simulink model "6DOF_model_2"  (R2019b)
settings: Solver=VariableStepAuto  StartTime=0.0  StopTime=10.0  RelTol=1e-3
values from neighbouring files (symbols this model uses):
  altitude = 0    [runFrist.m]
  AR = b^2/S    (= 7.81468427964)    [runFrist.m]
  b = 1.4224    [runFrist.m]
  c_bar = 0.3302    [runFrist.m]
  CDdelta_e = 0    [runFrist.m]
  Cdo = 0.03    [runFrist.m]
  CDq = 0    [runFrist.m]
  Clbeta = -0.12    [runFrist.m]
  Cldelta_a = 0.08    [runFrist.m]
  CLdelta_e = -0.36    [runFrist.m]
  Cldelta_r = 0.105    [runFrist.m]
  Clo = 0    [runFrist.m]
  Clp = -0.26    [runFrist.m]
  CLq = 0    [runFrist.m]
  Clr = 0.14    [runFrist.m]
  Cmalpha = -0.38    [runFrist.m]
  Cmdelta_e = -0.5    [runFrist.m]
  Cmo = 0    [runFrist.m]
  Cmq = -3.6    [runFrist.m]
  Cnbeta = 0.25    [runFrist.m]
  Cndelta_a = 0.06    [runFrist.m]
  Cndelta_r = -0.032    [runFrist.m]
  Cno = 0    [runFrist.m]
  Cnp = 0.022    [runFrist.m]
  Cnr = -0.35    [runFrist.m]
  Cybeta = -0.98    [runFrist.m]
  Cydelta_a = 0    [runFrist.m]
  Cydelta_r = -0.17    [runFrist.m]
  Cyo = 0    [runFrist.m]
  Cyp = 0    [runFrist.m]
  Cyr = 0    [runFrist.m]
  delta = Iz*Ix-Ixz^2    (= 196.36639775)    [runFrist.m]
  g = 9.81    [runFrist.m]
  I1 = Ixz*(Ix-Iy+Iz)    (= 2.56808565)    [runFrist.m]
  I2 = Iy*Iz-Iz^2-Ixz^2    (= -2930845.3888)    [runFrist.m]
  I3 = Ixz^2-Iy*Ix+Ix^2    (= 0.00655162)    [runFrist.m]
  Ix = 0.1147    [runFrist.m]
  Ixz = 0.0015    [runFrist.m]
  Iy = 0.0576    [runFrist.m]
  Iz = 01712    (= 1712)    [runFrist.m]
  m = 1.56    [runFrist.m]
  S = 0.2589    [runFrist.m]
  Thrust = 10    [runFrist.m]
  Uo = 0.01    [runFrist.m]
settings Model: Creator=Tinash  LastModifiedBy=Tinash

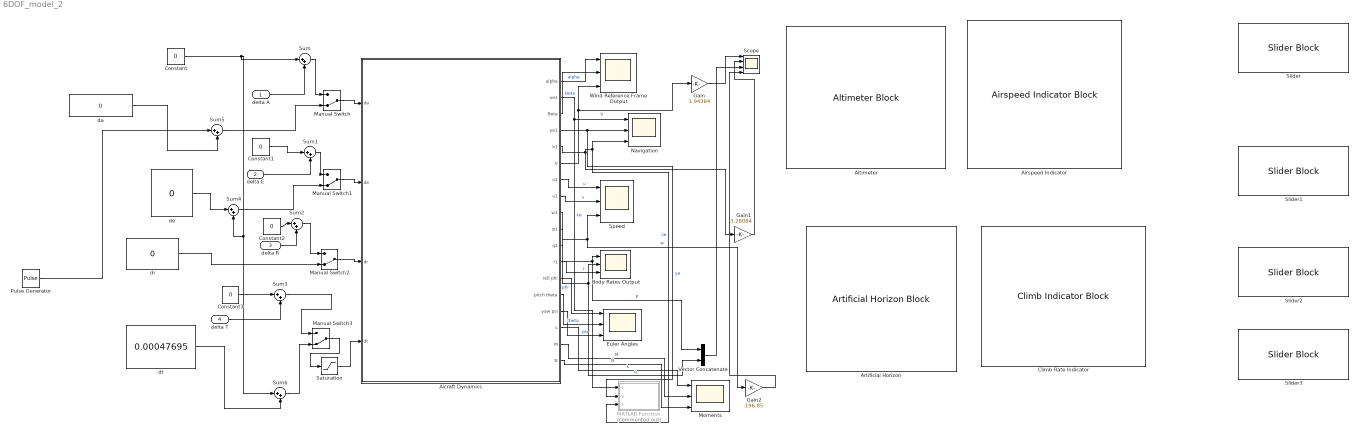
== system 6DOF_model_2 ==
  delta A : Inport
  delta E : Inport  Port=2
  delta R : Inport  Port=3
  delta T : Inport  Port=4
  Aicraft Dynamics : Subsystem
  Airspeed Indicator : AirspeedIndicatorBlock  BlockKeywords=__PRM__SERIALIZED__DATA__:flight instrument,gauge,cockpit,measurement,display,graphics,visualization,dashboard,aircraft,needle,instrumentation,speed,stall speed,maximum speed,max speed,ASI  ScaleMin=0  ScaleMax=100
  Altimeter : AltimeterBlock  BlockKeywords=__PRM__SERIALIZED__DATA__:flight instrument,gauge,cockpit,measurement,indicator,display,graphics,visualization,dashboard,aircraft,needle,instrumentation,altitude,height,height above sea level,altimetry,pressure altitude,atmospheric pressure
  Artificial Horizon : ArtificialHorizonBlock  BlockKeywords=__PRM__SERIALIZED__DATA__:flight instrument,gauge,cockpit,measurement,indicator,display,graphics,visualization,dashboard,aircraft,instrumentation,roll,pitch,attitude,angle,gyro horizon,gyroscope
  Body Rates Output : Scope  NumInputPorts=3
  Climb Rate Indicator : ClimbIndicatorBlock  BlockKeywords=__PRM__SERIALIZED__DATA__:flight instrument,gauge,cockpit,measurement,indicator,display,graphics,visualization,dashboard,aircraft,needle,instrumentation,climb indicator,altitude,sink rate,rate of descent,rate of ascent,vertical speed,variometer,vertical speed indicator,VSI,vertical velocity indicator,VVI,RCDI
  Constant{,1..3} (4 alike) : Constant  Value=0
  Euler Angles : Scope  NumInputPorts=3
  Gain : Gain  Gain=1.94384
  Gain1 : Gain  Gain=3.28084
  Gain2 : Gain  Gain=196.85
  MATLAB Function : MATLAB Function  Commented=on  TreatAsAtomicUnit=on
  Manual Switch{,1..3} (4 alike) : ManualSwitch  CurrentSetting=0
  Moments : Scope  NumInputPorts=3
  Navigation : Scope  NumInputPorts=3
  Pulse Generator : DiscretePulseGenerator  PulseType=Time based  Amplitude=0.1
  Saturation : Saturate  UpperLimit=inf  LowerLimit=-inf
  Scope : Scope  NumInputPorts=4
  Slider : SliderBlock  ScaleMin=-10  ScaleMax=10
  Slider1 : SliderBlock  ScaleMin=-10  ScaleMax=10
  Slider2 : SliderBlock  ScaleMin=-10  ScaleMax=10
  Slider3 : SliderBlock
  Speed : Scope  NumInputPorts=3
  Sum{,1..6} (7 alike) : Sum  Inputs=|++
  Vector Concatenate : Concatenate
  "Wind Reference Frame Output " : Scope  NumInputPorts=3
  da : Constant  Value=0
  de : Constant  Value=0
  dr : Constant  Value=0
  dt : Constant  Value=0.00047695  VectorParams1D=off
  wires:
  Saturation/1 -> Aicraft Dynamics/4(dt)
  Pulse Generator/1 -> Sum5/1
  Aicraft Dynamics/8(v1) -> Speed/2  "v"
  da/1 -> Sum5/2
  de/1 -> Sum4/1
  dt/1 -> Sum6/2
  Constant1/1 -> Sum1/1
  Manual Switch/1 -> Aicraft Dynamics/1(da)
  Sum3/1 -> Manual Switch3/1
  Sum4/1 -> Manual Switch1/2
  Aicraft Dynamics/3(Beta) -> "Wind Reference Frame Output "/2  "Beta"
  Aicraft Dynamics/12(r1) -> Body Rates Output/3  "r"
  Sum2/1 -> Manual Switch2/1
  Constant2/1 -> Sum2/1
  delta T/1 -> Sum3/2
  Sum6/1 -> Manual Switch3/2
  Sum/1 -> Manual Switch/1
  Sum5/1 -> Manual Switch/2
  Aicraft Dynamics/4(ye1) -> MATLAB Function/2(y), Navigation/2  "ye"
  Manual Switch3/1 -> Saturation/1
  Aicraft Dynamics/11(q1) -> Body Rates Output/2, Vector Concatenate/2  "q"
  Manual Switch2/1 -> Aicraft Dynamics/3(dr)
  Constant/1 -> Sum4/2, Sum6/1, Sum/1
  Aicraft Dynamics/9(w1) -> Speed/3, Gain2/1  "w"
  Aicraft Dynamics/10(p1) -> Body Rates Output/1, Vector Concatenate/1  "p"
  delta E/1 -> Sum1/2
  Aicraft Dynamics/15(yaw psi) -> Euler Angles/3  "psi"
  Manual Switch1/1 -> Aicraft Dynamics/2(de)
  Constant3/1 -> Sum3/1
  Aicraft Dynamics/7(u1) -> Speed/1  "u"
  Gain2/1 -> Scope/4
  dr/1 -> Manual Switch2/2
  delta R/1 -> Sum2/2
  Aicraft Dynamics/2(xe1) -> MATLAB Function/1(x), Navigation/1  "xe"
  delta A/1 -> Sum/2
  Aicraft Dynamics/6(V) -> Gain/1, "Wind Reference Frame Output "/3  "V"
  Aicraft Dynamics/1(alpha) -> "Wind Reference Frame Output "/1  "alpha"
  Sum1/1 -> Manual Switch1/1
  Aicraft Dynamics/13(roll phi) -> Euler Angles/1  "phi"
  Aicraft Dynamics/5(h1) -> MATLAB Function/3(z), Navigation/3, Gain1/1  "ze"
  Vector Concatenate/1 -> Scope/3
  Gain/1 -> Scope/1
  Gain1/1 -> Scope/2
  Aicraft Dynamics/14(pitch theta) -> Euler Angles/2  "theta"
  Aicraft Dynamics/16(L) -> Moments/1  "L"
  Aicraft Dynamics/17(M) -> Moments/2  "M"
  Aicraft Dynamics/18(N) -> Moments/3  "N"

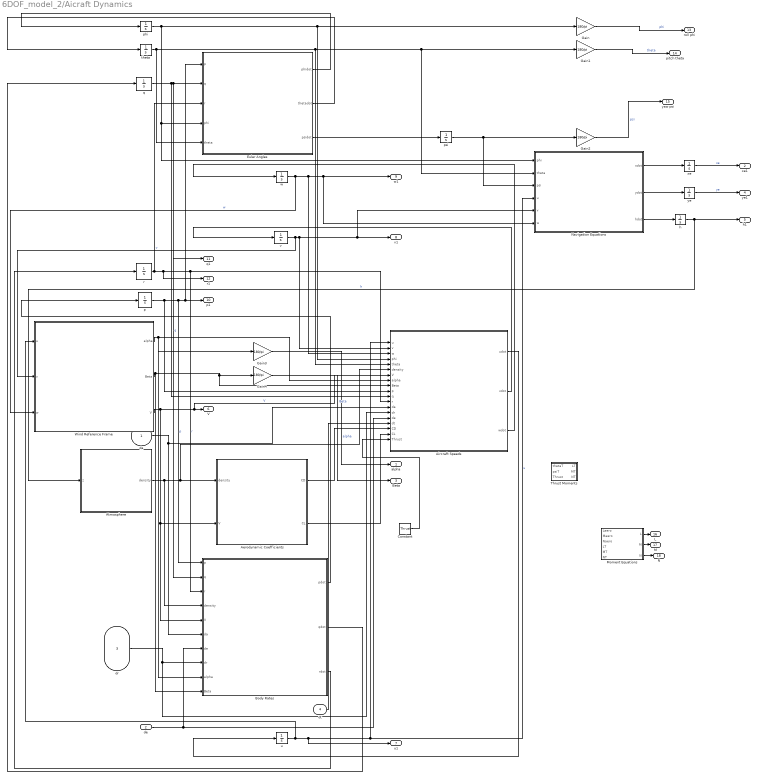
== system 6DOF_model_2/Aicraft Dynamics ==
  da : Inport
  de : Inport  Port=2
  dr : Inport  Port=3
  dt : Inport  Port=4
  Aerodynamic Coefficients : MATLAB Function  TreatAsAtomicUnit=on
  Aircraft Speeds : MATLAB Function  TreatAsAtomicUnit=on
  Atmosphere : MATLAB Function  TreatAsAtomicUnit=on
  Body Rates : MATLAB Function  TreatAsAtomicUnit=on
  Constant : Constant  Value=Thrust
  Euler Angles : MATLAB Function  TreatAsAtomicUnit=on
  Gain{,1..4} (5 alike) : Gain  Gain=180/pi
  Moment Equations : MATLAB Function  TreatAsAtomicUnit=on
  Navigation Equations : MATLAB Function  TreatAsAtomicUnit=on
  Thrust Moments : MATLAB Function  TreatAsAtomicUnit=on
  Wind Reference Frame : MATLAB Function  TreatAsAtomicUnit=on
  h : Integrator  InitialCondition=altitude  LimitOutput=on  LowerSaturationLimit=0
  p : Integrator
  phi : Integrator  LimitOutput=on  UpperSaturationLimit=2*pi  LowerSaturationLimit=0
  psi : Integrator  LimitOutput=on  UpperSaturationLimit=2*pi  LowerSaturationLimit=0
  q : Integrator
  r : Integrator
  theta : Integrator  LimitOutput=on  UpperSaturationLimit=0.9999*(pi/2)  LowerSaturationLimit=-0.99999*(pi/2)
  u : Integrator  InitialCondition=Uo  LimitOutput=on  LowerSaturationLimit=0.000000001
  v : Integrator
  w : Integrator
  xe : Integrator
  ye : Integrator
  alpha : Outport
  xe1 : Outport  Port=2
  Beta : Outport  Port=3
  ye1 : Outport  Port=4
  h1 : Outport  Port=5
  V : Outport  Port=6
  u1 : Outport  Port=7
  v1 : Outport  Port=8
  w1 : Outport  Port=9
  p1 : Outport  Port=10
  q1 : Outport  Port=11
  r1 : Outport  Port=12
  roll phi : Outport  Port=13
  pitch theta : Outport  Port=14
  yaw psi : Outport  Port=15
  L : Outport  Port=16
  M : Outport  Port=17
  N : Outport  Port=18
  wires:
  Gain4/1 -> Beta/1  "Beta"
  q/1 -> Euler Angles/2(q), q1/1, Body Rates/2(q), Aircraft Speeds/11(q)  "q"
  ye/1 -> ye1/1  "ye"
  r/1 -> Body Rates/3(r), Aircraft Speeds/12(r), r1/1, Euler Angles/3(r)  "r"
  Gain3/1 -> alpha/1  "alpha"
  xe/1 -> xe1/1  "xe"
  Body Rates/3(rdot) -> r/1
  Body Rates/2(qdot) -> q/1
  Euler Angles/3(psidot) -> psi/1
  Aircraft Speeds/3(wdot) -> w/1
  Euler Angles/2(thetadot) -> theta/1
  v/1 -> Navigation Equations/5(v), v1/1, Aircraft Speeds/2(v), Wind Reference Frame/2(v)  "v"
  Euler Angles/1(phidot) -> phi/1
  Body Rates/1(pdot) -> p/1
  Wind Reference Frame/1(alpha) -> Gain3/1, Aircraft Speeds/8(alpha), Body Rates/9(alpha)
  Aerodynamic Coefficients/2(CL) -> Aircraft Speeds/18(CL)
  dt/1 -> Aircraft Speeds/16(dt)
  Navigation Equations/2(ydot) -> ye/1
  theta/1 -> Navigation Equations/2(theta), Gain1/1, Aircraft Speeds/5(theta), Euler Angles/5(theta)
  psi/1 -> Gain2/1, Navigation Equations/3(psi)
  phi/1 -> Navigation Equations/1(phi), Euler Angles/4(phi), Aircraft Speeds/4(phi), Gain/1
  Navigation Equations/1(xdot) -> xe/1
  Aircraft Speeds/2(vdot) -> v/1
  Aircraft Speeds/1(udot) -> u/1
  Aerodynamic Coefficients/1(CD) -> Aircraft Speeds/17(CD)
  Navigation Equations/3(hdot) -> h/1
  da/1 -> Body Rates/6(da), Aircraft Speeds/13(da)
  w/1 -> Navigation Equations/6(w), w1/1, Aircraft Speeds/3(w), Wind Reference Frame/3(w)  "w"
  p/1 -> Euler Angles/1(p), p1/1, Body Rates/1(p), Aircraft Speeds/10(p)  "p"
  u/1 -> Aircraft Speeds/1(u), Navigation Equations/4(u), u1/1, Wind Reference Frame/1(u)  "u"
  h/1 -> Atmosphere/1(z), h1/1  "h"
  de/1 -> Body Rates/7(de), Aircraft Speeds/15(de)
  dr/1 -> Aircraft Speeds/14(dr), Body Rates/8(dr)
  Atmosphere/1(density) -> Aircraft Speeds/6(density), Aerodynamic Coefficients/1(density), Body Rates/4(density)
  Wind Reference Frame/3(V) -> Body Rates/5(V), Aerodynamic Coefficients/2(V), Aircraft Speeds/7(V), V/1  "V"
  Wind Reference Frame/2(Beta) -> Gain4/1, Aircraft Speeds/9(Beta), Body Rates/10(Beta)
  Gain/1 -> roll phi/1  "phi"
  Gain1/1 -> pitch theta/1  "theta"
  Gain2/1 -> yaw psi/1  "psi"
  Constant/1 -> Aircraft Speeds/19(Thrust)
  Moment Equations/1(L) -> L/1
  Moment Equations/2(M) -> M/1
  Moment Equations/3(N) -> N/1

== matlab function 6DOF_model_2/Aicraft Dynamics/Aircraft Speeds ==
  data: u input; udot output size=1; vdot output size=1; wdot output size=1; v input; w input; phi input; theta input; g parameter; density input; V input; m parameter; alpha input; Beta input; Cybeta parameter; Cyo parameter; Cyp parameter; p input; q input; r input; b parameter; Cydelta_a parameter; da input; dr input; de input; dt input; Cydelta_r parameter; c_bar parameter; CD input; CDq parameter; CLq parameter; CDdelta_e parameter; CL input; CLdelta_e parameter; S parameter; Cyr parameter; Thrust input
function [udot,vdot,wdot] = fcn(u,v,w,phi,theta,g,density,V,m,...
    alpha,Beta,Cybeta, Cyo,Cyp,p,q,r,b,Cydelta_a,da,dr,de,dt,...
    Cydelta_r,c_bar,CD,CDq, CLq,...
    CDdelta_e, CL,CLdelta_e,S,Cyr,Thrust)
%Consider making CL dynamic
Cx=CD*cos(alpha)+CL*sin(alpha);
Cxq=-CDq*cos(alpha)+CLq*sin(alpha);
Cxde=-CDdelta_e*cos(alpha)+CLdelta_e*sin(alpha);
Cz=-CD*sin(alpha)-CL*cos(alpha);
Czq=-CDq*sin(alpha)-CLq*cos(alpha);
Czde=-CDdelta_e*sin(alpha)-CLdelta_e*cos(alpha);



udot=r*v - q*w -g*sin(theta)+ (density*V^2*S*0.5/m)*...
    (Cx + (Cxq*c_bar*q*0.5/m)+Cxde*de+...
    -(Thrust*g/m)*dt);


vdot=p*w-r*u+g*cos(theta)*sin(phi)+(density*V^2*S*0.5/m)*...
    (Cyo+Cybeta*Beta+Cyp*(b*p*0.5/V)+Cyr*(b*r*0.5/V)+Cydelta_a*da+...
    Cydelta_r*dr);

wdot=q*u-p*v+g*cos(theta)*cos(phi)+(density*V^2*S*0.5/m)*...
    (Cz+(Czq*c_bar*q*0.5/V)+Czde*de);


end

== matlab function 6DOF_model_2/Aicraft Dynamics/Navigation Equations ==
  data: phi input; theta input; psi input; u input; xdot output; v input; w input; ydot output; hdot output
function [xdot,ydot,hdot] = fcn(phi,theta,psi,u,v,w)
xdot=(cos(theta)*cos(psi))*u+...
    (sin(phi)*sin(theta)*cos(psi)-cos(phi)*sin(psi))*v+...
    (cos(phi)*sin(theta)*cos(psi)+sin(phi)*sin(psi))*w;

ydot=(cos(theta)*sin(psi))*u+...
    (sin(phi)*sin(theta)*cos(psi)+cos(phi)*sin(psi))*v...
    +(cos(phi)*sin(theta)*sin(psi)-sin(phi)*cos(psi))*w;

zdot=u*sin(theta)-v*sin(phi)*cos(theta)-w*cos(phi)*cos(theta);
hdot=-zdot;
end

== matlab function 6DOF_model_2/Aicraft Dynamics/Euler Angles ==
  data: p input; phidot output; thetadot output; psidot output; q input; r input; phi input; theta input
function [phidot,thetadot,psidot] = fcn(p,q,r,phi,theta)
phidot=p+q*sin(phi)*tan(theta)+r*cos(phi)*tan(theta);

thetadot=q*cos(phi)-r*sin(phi);

psidot=q*sin(phi)*sec(theta)+r*cos(phi)*sec(theta);





end

== matlab function 6DOF_model_2/Aicraft Dynamics/Body Rates ==
  data: p input; pdot output size=1; qdot output size=1; rdot output size=1; q input; r input; I1 parameter; I2 parameter; delta parameter; I3 parameter; Ix parameter; Iy parameter; Iz parameter; Ixz parameter; density input; V input; S parameter; b parameter; Clo parameter; Cno parameter; Clbeta parameter; Cnbeta parameter; Cnp parameter; Clp parameter; Clr parameter; Cnr parameter; da input; de input; dr input; Cldelta_r parameter; Cldelta_a parameter; Cndelta_r parameter; Cndelta_a parameter; alpha input; Cmalpha parameter; Cmdelta_e parameter; Cmo parameter; c_bar parameter; Beta input; Cmq parameter
function [pdot,qdot,rdot] = fcn(p,q,r,I1, I2, delta, I3, Ix, Iy, Iz, Ixz...
    ,density,V,S, b,Clo, Cno,Clbeta,Cnbeta,Cnp,Clp,Clr, Cnr,...
    da,de,dr,Cldelta_r,Cldelta_a, Cndelta_r, Cndelta_a,...
    alpha, Cmalpha,Cmdelta_e, Cmo, c_bar,Beta,Cmq)
 
Cpo=(Iz*Clo/delta)+(Ixz*Cno/delta);
CpBeta=(Iz*Clbeta/delta)+(Ixz*Cnbeta/delta);
Cpr=(Iz*Clr/delta)+(Ixz*Cnr/delta);
Cpda=(Iz*Cldelta_a/delta)+(Ixz*Cndelta_a/delta);
Cpdr=(Iz*Cldelta_r/delta)+(Ixz*Cndelta_r/delta);
Cpp=(Iz*Clp/delta)+(Ixz*Cnp/delta);

Cro=(Ixz*Clo/delta) + (Ix*Cno/delta);
CrBeta=(Ixz*Clbeta/delta) + (Ix*Cnbeta/delta);
Crp=(Ixz*Clp/delta) + (Ix*Cnp/delta);
Crr=(Ixz*Clr/delta) + (Ix*Cnr/delta);
Crda=(Ixz*Cldelta_a/delta) + (Ix*Cndelta_a/delta);
Crdr=(Ixz*Cldelta_r/delta) + (Ix*Cndelta_r/delta);
%-----------------------------------------
pdot=(I1*p*q/delta)+ (I2*q*r/delta) + (0.5*density*V^2*S*b)*...
    (Cpo+CpBeta*Beta +(Cpp*b*p*0.5/V)+(Cpr*b*r*0.5/V)+Cpda*da+Cpdr*dr);


qdot=((Iz-Ix)*p*r/delta)-(Ixz*(p^2-r^2)/delta)+(0.5*density*V^2*S*c_bar/Iy)...
    *(Cmo+Cmalpha*alpha+Cmq*(c_bar*q*0.5/V)+Cmdelta_e*de);


rdot=(I3*p*q/delta) - (I1*q*r/delta) + (0.5*density*V^2*S*b)*...
    (Cro +CrBeta*Beta + (Crp*b*p*0.5/V) + (Crr*b*r*0.5/V)+ ...
    Crda*da + Crdr*dr);

end

== matlab function 6DOF_model_2/Aicraft Dynamics/Wind Reference Frame ==
  data: u input; alpha output size=1; Beta output size=1; V output size=1; v input; w input
function [alpha,Beta,V] = fcn(u,v,w)
V=sqrt(u^2+v^2+w^2);

alpha=atan(w/u);

Beta=atan(v/sqrt(u^2+w^2))
end

== matlab function 6DOF_model_2/Aicraft Dynamics/Atmosphere ==
  data: z input; density output
function density  = fcn(z)
density=1.225;
h=abs(z);
h=0.3048*h;%if working in ft
%--------------------------
if h>=25000
    T=-131.21+0.00299*h
    P=2.488*((T+273.1)/216.6)^-11.388;
     density=P/(0.2869*(T+273.1));

%----------------------------

%-------------------------------
elseif (11000<h)&&(h<25000)
    T=-56.46;
    P=22.65*exp(1.73-0.000157*h);
     density=P/(0.2869*(T+273.1));

%---------------------------------   

%-----------------------------------
elseif h<=11000
       T=15.04-0.00649*h;
       P=101.29*((T+273.1)/288.08)^5.256;
       density=P/(0.2869*(T+273.1));
else
    density=1.225;
 %----------------------------------
 density =0.0624279606*density; 

end

== matlab function 6DOF_model_2/Aicraft Dynamics/Aerodynamic Coefficients ==
  data: CD output size=1; AR parameter; e parameter; Cdo parameter; density input; V input; CL output size=1; m parameter; S parameter; g parameter
function [CD,CL] = fcn(AR, e,Cdo,density,V,m, S, g)

CL=(2*m*g)/(density*V^2*S);

CD=Cdo +CL^2/(AR*e*pi)

end

== matlab function 6DOF_model_2/MATLAB Function ==
  data: x input; y input; z input
function fcn(x,y,z)
plot3(x,y,z);
hold on;
end

== matlab function 6DOF_model_2/Aicraft Dynamics/Moment Equations ==
  data: Laero input; L output; M output; N output; Maero input; Naero input; LT input; MT input; NT input
function [L,M,N] = fcn(Laero,Maero,Naero,LT,MT,NT)

end

== matlab function 6DOF_model_2/Aicraft Dynamics/Thrust Moments ==
  data: thetaT input; LT output; psiT input; MT output; NT output; Thrust input
function [LT,MT,NT] = fcn(thetaT,psiT,Thrust)
%to be worked on
T=Thrust;
LT=0;
YT=0;
NT=0;



end
